simulink library "Kitchen_Lib"  (R2023a)
settings: Solver=VariableStepAuto  StartTime=0.0  StopTime=10.0  RelTol=1e-3  EnableMultiTasking=on
undefined symbols (not defined in the file): Kitc_BusTyp_P, Kitc_BusTypSkyr_C, Kitc_ColrLedColrls_C, Kitc_ColrLedGrn_C, Kitc_ColrLedRed_C, Kitc_ColrLedYlw_C, Kitc_StDgnWtrTank_C, Kitc_StElecPlugScktOffByClmp50_P, Kitc_StsDlyBlink_C, Kitc_StsErrBlink_C, Kitc_StsFctAcvn_P, Kitc_StsInfoBlink_C, Kitc_StsKitchnOffAutoIgOff_P, Kitc_StsKitchnOffBySwt_P, Kitc_StsKitchnOffDoorLockd_P, Kitc_StsKitchnOffIgOff_P, Kitc_StsKitchnOffUv_P, Kitc_StsKitchnOnBySwt_P, Kitc_StsKitchnOnNVM_P, Kitc_StsLedOff_C, Kitc_StsLedOn_C, Kitc_StsLrgCnsAcv_P, Kitc_StTrfrAnSwtInstd_P, Kitc_StTrfrSwtInstd_P, Kitc_TiKitcRefgtrOffDly_P, Kitc_ULowrThdBat_C, Kitc_UUpprThdBat_C, Kitc_ValFalse_C, Kitc_ValPwmFreq2_C, Kitc_ValPwmFreq_C, Kitc_ValTrue_C
libraries: MAN_Library x50, E2E_Lib x3
(part 10 of 13)

== system Kitchen_Lib/Kitchen/100ms/Kitchn/Subsystem1/Subsystem19/Trfr/TurnOnDelay/TurnOnDelayOriginal/RisingEdgeDetection ==
  CLK : Inport
  Constant : Constant  Value=boolean(1)  OutDataTypeStr=boolean
  Data Type Conversion1 : DataTypeConversion  OutDataTypeStr=boolean  SaturateOnIntegerOverflow=off  RndMeth=Floor
  Logical Operator : Logic  AllPortsSameDT=off  OutDataTypeStr=boolean
  Relational Operator : RelationalOperator  Operator=~=  OutDataTypeStr=boolean  InputSameDT=off
  Relational Operator1 : RelationalOperator  Operator===  OutDataTypeStr=boolean  InputSameDT=off
  Unit Delay : UnitDelay  SampleTime=-1  HasFrameUpgradeWarning=on
  Q : Outport
  wires:
  Data Type Conversion1/1 -> Relational Operator1/1, Relational Operator/2, Unit Delay/1
  Constant/1 -> Relational Operator1/2
  Logical Operator/1 -> Q/1
  Relational Operator1/1 -> Logical Operator/2
  Relational Operator/1 -> Logical Operator/1
  Unit Delay/1 -> Relational Operator/1
  CLK/1 -> Data Type Conversion1/1

== system Kitchen_Lib/Kitchen/100ms/Kitchn/Subsystem1/Subsystem19/Trfr/TurnOnDelay/TurnOnDelayOriginal/TimePulseOriginal ==
  TimePulseEnable : Inport
  TimePulseDuration : Inport  Port=2
  CycleTime : Inport  Port=3
  Data Type Conversion1 : DataTypeConversion  OutDataTypeStr=uint32  SaturateOnIntegerOverflow=off  RndMeth=Floor
  Data Type Conversion2 : DataTypeConversion  OutDataTypeStr=boolean  SaturateOnIntegerOverflow=off  RndMeth=Floor
  Delay1 : Delay  DelayLength=1  InitialCondition=0  ExternalReset=Rising
      settings: InputPortMap=u0,r5
  Logical Operator1 : Logic  Operator=NOT  AllPortsSameDT=off  OutDataTypeStr=boolean
  Logical Operator2 : Logic  AllPortsSameDT=off  OutDataTypeStr=boolean
  RisingEdgeDetection : Subsystem  AncestorBlock=MAN_Library/RisingEdgeDetection
  RisingEdgeDetection1 : Subsystem  AncestorBlock=MAN_Library/RisingEdgeDetection
  SR : Subsystem  AncestorBlock=MAN_Library/SR
  TimerCountingUpOriginal : Subsystem  AncestorBlock=MAN_Library/BasicLibrary/TimerCountingUpOriginal
  TimePulseFlag : Outport
  TimePulseExpiredTime : Outport  Port=2
  wires:
  CycleTime/1 -> TimerCountingUpOriginal/4(CycleTime)
  Delay1/1 -> SR/2(R)
  [TimePulseReset] -> TimerCountingUpOriginal/2(TimerReset)
  [TimePulseReset] -> Delay1/2
  RisingEdgeDetection/1(Q) -> SR/1(S), [TimePulseReset]
  Data Type Conversion1/1 -> TimerCountingUpOriginal/3(TimerThreshold)
  Data Type Conversion2/1 -> RisingEdgeDetection/1(CLK)
  Logical Operator1/1 -> Logical Operator2/2
  Logical Operator2/1 -> TimePulseFlag/1
  RisingEdgeDetection1/1(Q) -> Delay1/1
  TimerCountingUpOriginal/1(TimerFlag) -> RisingEdgeDetection1/1(CLK), Logical Operator1/1
  SR/1(Q) -> Logical Operator2/1, TimerCountingUpOriginal/1(TimerEnable)
  TimePulseEnable/1 -> Data Type Conversion2/1
  TimePulseDuration/1 -> Data Type Conversion1/1
  TimerCountingUpOriginal/2(TimerCurrentValue) -> TimePulseExpiredTime/1

== system Kitchen_Lib/Kitchen/100ms/Kitchn/Subsystem1/Subsystem19/WaterTankEmptyDiagnostic/Diagno sticsDebouncing/DiagnosticsDebouncingOriginal/RS ==
  S : Inport
  R : Inport  Port=2
  Constant2 : Constant  Value=boolean(1)  OutDataTypeStr=boolean
  Constant3 : Constant  Value=boolean(0)  OutDataTypeStr=boolean
  Data Type Conversion1 : DataTypeConversion  OutDataTypeStr=boolean  SaturateOnIntegerOverflow=off  RndMeth=Floor
  Data Type Conversion2 : DataTypeConversion  OutDataTypeStr=boolean  SaturateOnIntegerOverflow=off  RndMeth=Floor
  Multiport Switch : MultiPortSwitch  DataPortOrder=Zero-based contiguous  Inputs=2  zeroidx=on  SaturateOnIntegerOverflow=off  InputSameDT=off
  Multiport Switch2 : MultiPortSwitch  DataPortOrder=Zero-based contiguous  Inputs=2  zeroidx=on  SaturateOnIntegerOverflow=off  InputSameDT=off
  Unit Delay : UnitDelay  SampleTime=-1  HasFrameUpgradeWarning=on
  Q : Outport
  wires:
  Data Type Conversion1/1 -> Multiport Switch2/1
  Data Type Conversion2/1 -> Multiport Switch/1
  Multiport Switch2/1 -> Unit Delay/1, Q/1
  Multiport Switch/1 -> Multiport Switch2/2
  Constant3/1 -> Multiport Switch2/3
  R/1 -> Data Type Conversion1/1
  Unit Delay/1 -> Multiport Switch/2
  Constant2/1 -> Multiport Switch/3
  S/1 -> Data Type Conversion2/1

== system Kitchen_Lib/Kitchen/100ms/Kitchn/Subsystem1/Subsystem19/WaterTankEmptyDiagnostic/Diagno sticsDebouncing/DiagnosticsDebouncingOriginal/TurnOffDelayOriginal  ==
  TurnOffDelayEnable : Inport
  TurnOffDelayThreshold : Inport  Port=2
  CycleTime : Inport  Port=3
  Data Type Conversion1 : DataTypeConversion  OutDataTypeStr=uint32  SaturateOnIntegerOverflow=off  RndMeth=Floor
  Data Type Conversion2 : DataTypeConversion  OutDataTypeStr=boolean  SaturateOnIntegerOverflow=off  RndMeth=Floor
  Data Type Conversion3 : DataTypeConversion  OutDataTypeStr=uint32  SaturateOnIntegerOverflow=off  RndMeth=Floor
  FallingEdgeDetection : Subsystem  AncestorBlock=MAN_Library/FallingEdgeDetection
  Logical Operator2 : Logic  Operator=OR  AllPortsSameDT=off  OutDataTypeStr=boolean
  TimePulseOriginal : Subsystem  AncestorBlock=MAN_Library/BasicLibrary/TimePulseOriginal
  TurnOffDelayFlag : Outport
  TurnOffDelayExpiredTime : Outport  Port=2
  wires:
  CycleTime/1 -> TimePulseOriginal/3(CycleTime)
  Data Type Conversion3/1 -> TurnOffDelayExpiredTime/1
  Data Type Conversion1/1 -> TimePulseOriginal/2(TimePulseDuration)
  TurnOffDelayThreshold/1 -> Data Type Conversion1/1
  FallingEdgeDetection/1(Q) -> TimePulseOriginal/1(TimePulseEnable)
  TimePulseOriginal/2(TimePulseExpiredTime) -> Data Type Conversion3/1
  Logical Operator2/1 -> TurnOffDelayFlag/1
  TimePulseOriginal/1(TimePulseFlag) -> Logical Operator2/2
  Data Type Conversion2/1 -> FallingEdgeDetection/1(CLK), Logical Operator2/1
  TurnOffDelayEnable/1 -> Data Type Conversion2/1

== system Kitchen_Lib/Kitchen/100ms/Kitchn/Subsystem1/Subsystem19/WaterTankEmptyDiagnostic/Diagno sticsDebouncing/DiagnosticsDebouncingOriginal/TurnOnDelayOriginal ==
  TurnOnDelayEnable : Inport
  TurnOnDelayThreshold : Inport  Port=2
  CycleTime : Inport  Port=3
  Data Type Conversion1 : DataTypeConversion  OutDataTypeStr=uint32  SaturateOnIntegerOverflow=off  RndMeth=Floor
  Data Type Conversion2 : DataTypeConversion  OutDataTypeStr=boolean  SaturateOnIntegerOverflow=off  RndMeth=Floor
  Logical Operator1 : Logic  Operator=NOT  AllPortsSameDT=off  OutDataTypeStr=boolean
  Logical Operator2 : Logic  AllPortsSameDT=off  OutDataTypeStr=boolean
  RisingEdgeDetection : Subsystem  AncestorBlock=MAN_Library/RisingEdgeDetection
  TimePulseOriginal : Subsystem  AncestorBlock=MAN_Library/BasicLibrary/TimePulseOriginal
  TurnOnDelayFlag : Outport
  TurnOnDelayExpiredTime : Outport  Port=2
  wires:
  CycleTime/1 -> TimePulseOriginal/3(CycleTime)
  Logical Operator2/1 -> TurnOnDelayFlag/1
  TimePulseOriginal/1(TimePulseFlag) -> Logical Operator1/1
  Logical Operator1/1 -> Logical Operator2/2
  TimePulseOriginal/2(TimePulseExpiredTime) -> TurnOnDelayExpiredTime/1
  RisingEdgeDetection/1(Q) -> TimePulseOriginal/1(TimePulseEnable)
  Data Type Conversion1/1 -> TimePulseOriginal/2(TimePulseDuration)
  TurnOnDelayThreshold/1 -> Data Type Conversion1/1
  TurnOnDelayEnable/1 -> Data Type Conversion2/1
  Data Type Conversion2/1 -> RisingEdgeDetection/1(CLK), Logical Operator2/1

== system Kitchen_Lib/Kitchen/100ms/Kitchn/Subsystem1/Subsystem19/WaterTankEmptyDiagnostic/TurnOffDelay/TurnOffDelayOriginal/FallingEdgeDetection ==
  CLK : Inport
  Constant : Constant  Value=boolean(0)  OutDataTypeStr=boolean
  Data Type Conversion1 : DataTypeConversion  OutDataTypeStr=boolean  SaturateOnIntegerOverflow=off  RndMeth=Floor
  Logical Operator1 : Logic  AllPortsSameDT=off  OutDataTypeStr=boolean
  Relational Operator2 : RelationalOperator  Operator=~=  OutDataTypeStr=boolean  InputSameDT=off
  Relational Operator3 : RelationalOperator  Operator===  OutDataTypeStr=boolean  InputSameDT=off
  Unit Delay1 : UnitDelay  SampleTime=-1  HasFrameUpgradeWarning=on
  Q : Outport
  wires:
  Data Type Conversion1/1 -> Unit Delay1/1, Relational Operator2/2, Relational Operator3/1
  Constant/1 -> Relational Operator3/2
  CLK/1 -> Data Type Conversion1/1
  Logical Operator1/1 -> Q/1
  Relational Operator3/1 -> Logical Operator1/2
  Relational Operator2/1 -> Logical Operator1/1
  Unit Delay1/1 -> Relational Operator2/1

== system Kitchen_Lib/Kitchen/100ms/Kitchn/Subsystem1/Subsystem19/WaterTankEmptyDiagnostic/TurnOffDelay/TurnOffDelayOriginal/TimePulseOriginal ==
  TimePulseEnable : Inport
  TimePulseDuration : Inport  Port=2
  CycleTime : Inport  Port=3
  Data Type Conversion1 : DataTypeConversion  OutDataTypeStr=uint32  SaturateOnIntegerOverflow=off  RndMeth=Floor
  Data Type Conversion2 : DataTypeConversion  OutDataTypeStr=boolean  SaturateOnIntegerOverflow=off  RndMeth=Floor
  Delay1 : Delay  DelayLength=1  InitialCondition=0  ExternalReset=Rising
      settings: InputPortMap=u0,r5
  Logical Operator1 : Logic  Operator=NOT  AllPortsSameDT=off  OutDataTypeStr=boolean
  Logical Operator2 : Logic  AllPortsSameDT=off  OutDataTypeStr=boolean
  RisingEdgeDetection : Subsystem  AncestorBlock=MAN_Library/RisingEdgeDetection
  RisingEdgeDetection1 : Subsystem  AncestorBlock=MAN_Library/RisingEdgeDetection
  SR : Subsystem  AncestorBlock=MAN_Library/SR
  TimerCountingUpOriginal : Subsystem  AncestorBlock=MAN_Library/BasicLibrary/TimerCountingUpOriginal
  TimePulseFlag : Outport
  TimePulseExpiredTime : Outport  Port=2
  wires:
  CycleTime/1 -> TimerCountingUpOriginal/4(CycleTime)
  Delay1/1 -> SR/2(R)
  [TimePulseReset] -> TimerCountingUpOriginal/2(TimerReset)
  [TimePulseReset] -> Delay1/2
  RisingEdgeDetection/1(Q) -> SR/1(S), [TimePulseReset]
  Data Type Conversion1/1 -> TimerCountingUpOriginal/3(TimerThreshold)
  Data Type Conversion2/1 -> RisingEdgeDetection/1(CLK)
  Logical Operator1/1 -> Logical Operator2/2
  Logical Operator2/1 -> TimePulseFlag/1
  RisingEdgeDetection1/1(Q) -> Delay1/1
  TimerCountingUpOriginal/1(TimerFlag) -> RisingEdgeDetection1/1(CLK), Logical Operator1/1
  SR/1(Q) -> Logical Operator2/1, TimerCountingUpOriginal/1(TimerEnable)
  TimePulseEnable/1 -> Data Type Conversion2/1
  TimePulseDuration/1 -> Data Type Conversion1/1
  TimerCountingUpOriginal/2(TimerCurrentValue) -> TimePulseExpiredTime/1

== system Kitchen_Lib/Kitchen/100ms/Kitchn/Subsystem1/Subsystem16/001_KitchnCtl/002_FlipFlop/KSW-KitchenControl/KSW_Battery/BatteryVoltageUnder22.7V ==
  Kitchn_On : Inport
  EngOrAddlBat : Inport  Port=2
  "GW_Ubat " : Inport  Port=3
  Constant : Constant  Value=Kitc_StsLrgCnsAcv_P
  Constant2 : Constant  Value=Kitc_ULowrThdBat_C
  Data Store Read : DataStoreRead  DataStoreName=Kitc_StsLrgCnsAcvNv  IndexOptions=Index vector (dialog)  Indices=1  OutputSizes=1
  Data Type Conversion : DataTypeConversion  OutDataTypeStr=boolean  SaturateOnIntegerOverflow=off  RndMeth=Floor
  Logical Operator1 : Logic  Operator=NOT  Inputs=4  AllPortsSameDT=off  OutDataTypeStr=boolean
  Logical Operator2 : Logic  Inputs=4  AllPortsSameDT=off  OutDataTypeStr=boolean
  Relational Operator1 : RelationalOperator  Operator=<=  OutDataTypeStr=boolean  InputSameDT=off
  Switch : Switch  Criteria=u2 ~= 0  SaturateOnIntegerOverflow=off  InputSameDT=off
  BatUUnder22.7V : Outport
  wires:
  Data Type Conversion/1 -> Switch/2
  Constant/1 -> Switch/3
  Data Store Read/1 -> Switch/1, Data Type Conversion/1
  Logical Operator2/1 -> BatUUnder22.7V/1
  EngOrAddlBat/1 -> Logical Operator1/1
  "GW_Ubat "/1 -> Relational Operator1/1
  Constant2/1 -> Relational Operator1/2
  Relational Operator1/1 -> Logical Operator2/4
  Logical Operator1/1 -> Logical Operator2/1
  Switch/1 -> Logical Operator2/3
  Kitchn_On/1 -> Logical Operator2/2

== system Kitchen_Lib/Kitchen/100ms/Kitchn/Subsystem1/Subsystem16/001_KitchnCtl/002_FlipFlop/KSW-KitchenControl/KSW_Battery/BatteryVoltageUnder23V ==
  GW_Ubat : Inport
  EngOrAddlBat : Inport  Port=2
  Kitchn_On : Inport  Port=3
  Kitc_StsHostsCallAcv : Inport  Port=4
  Constant : Constant  Value=Kitc_StsLrgCnsAcv_P
  Constant1 : Constant  Value=Kitc_UUpprThdBat_C
  "Constant3  " : MAN_Library/TimeConstant  hours=0  minutes=0  seconds=10  miliseconds=0
  "Constant4  " : MAN_Library/TimeConstant  hours=0  minutes=10  seconds=0  miliseconds=0
  "Constant6  " : MAN_Library/TimeConstant  hours=0  minutes=0  seconds=0  miliseconds=500
  Data Store Read : DataStoreRead  DataStoreName=Kitc_StsLrgCnsAcvNv  IndexOptions=Index vector (dialog)  Indices=1  OutputSizes=1
  Data Type Conversion : DataTypeConversion  OutDataTypeStr=boolean  SaturateOnIntegerOverflow=off  RndMeth=Floor
  Logical Operator15 : Logic  Operator=OR  AllPortsSameDT=off  OutDataTypeStr=boolean
  Logical Operator16 : Logic  Operator=NOT  Inputs=4  AllPortsSameDT=off  OutDataTypeStr=boolean
  Logical Operator3 : Logic  Inputs=4  AllPortsSameDT=off  OutDataTypeStr=boolean
  Logical Operator4 : Logic  Operator=NOT  Inputs=4  AllPortsSameDT=off  OutDataTypeStr=boolean
  Relational Operator : RelationalOperator  Operator=<=  OutDataTypeStr=boolean  InputSameDT=off
  Switch : Switch  Criteria=u2 ~= 0  SaturateOnIntegerOverflow=off  InputSameDT=off
  Terminator : Terminator
  Terminator1 : Terminator
  Terminator2 : Terminator
  TimePulse : MAN_Library/TimePulse  CycleTime=Cycle Time: 10 Ms
  TimePulse1 : MAN_Library/TimePulse  CycleTime=Cycle Time: 10 Ms
  TurnOffDelay : MAN_Library/TurnOffDelay  CycleTime=Cycle Time: 10 Ms
  LrgCnsOff : Outport
  Kitc_WarnLrgCns : Outport  Port=2
  Kitc_StBuzRe : Outport  Port=3
  wires:
  Data Type Conversion/1 -> Switch/2
  Constant/1 -> Switch/3
  Data Store Read/1 -> Switch/1, Data Type Conversion/1
  Switch/1 -> Logical Operator3/3
  Constant1/1 -> Relational Operator/2
  Relational Operator/1 -> Logical Operator3/4
  Kitchn_On/1 -> Logical Operator3/2
  Logical Operator16/1 -> Logical Operator3/1
  EngOrAddlBat/1 -> Logical Operator16/1
  GW_Ubat/1 -> Relational Operator/1
  "Constant3  "/1 -> TimePulse/2
  TimePulse/1 -> Kitc_WarnLrgCns/1, Logical Operator15/1
  "Constant4  "/1 -> TurnOffDelay/2
  Logical Operator4/1 -> TurnOffDelay/1
  TurnOffDelay/1 -> LrgCnsOff/1
  Kitc_StsHostsCallAcv/1 -> TimePulse1/1
  Logical Operator15/1 -> Kitc_StBuzRe/1
  "Constant6  "/1 -> TimePulse1/2
  TimePulse1/1 -> Logical Operator15/2
  TurnOffDelay/2 -> Terminator/1
  TimePulse/2 -> Terminator1/1
  TimePulse1/2 -> Terminator2/1
  Logical Operator3/1 -> Logical Operator4/1, TimePulse/1

== system Kitchen_Lib/Kitchen/100ms/Kitchn/Subsystem1/Subsystem16/001_KitchnCtl/002_FlipFlop/KSW-KitchenControl/KSW_Battery/KitchenActivation ==
  note: Large Comsp
  "GW_StClmp50Off3Sec " : Inport
  "GW_StUvTopPrio " : Inport  Port=2
  "GW_ModeExbn " : Inport  Port=3
  CLS_StDoorLockdOutd : Inport  Port=4
  BatUUnder22.7V : Inport  Port=5
  LrgCnsOff : Inport  Port=6
  Kitchn_On : Inport  Port=7
  GW_StClmp15 : Inport  Port=8
  EngOrAddlBat : Inport  Port=9
  Constant : Constant  Value=Kitc_StsLrgCnsAcv_P
  Data Store Read : DataStoreRead  DataStoreName=Kitc_StsLrgCnsAcvNv  IndexOptions=Index vector (dialog)  Indices=1  OutputSizes=1
  Data Type Conversion : DataTypeConversion  OutDataTypeStr=boolean  SaturateOnIntegerOverflow=off  RndMeth=Floor
  Logical Operator{1,9..12} (5 alike) : Logic  Operator=NOT  Inputs=4  AllPortsSameDT=off  OutDataTypeStr=boolean
  Logical Operator13 : Logic  Operator=OR  AllPortsSameDT=off  OutDataTypeStr=boolean
  Logical Operator14 : Logic  AllPortsSameDT=off  OutDataTypeStr=boolean
  Logical Operator5 : Logic  Operator=OR  AllPortsSameDT=off  OutDataTypeStr=boolean
  Logical Operator6 : Logic  Inputs=3  AllPortsSameDT=off  OutDataTypeStr=boolean
  Logical Operator7 : Logic  Inputs=9  AllPortsSameDT=off  OutDataTypeStr=boolean
  Switch : Switch  Criteria=u2 ~= 0  SaturateOnIntegerOverflow=off  InputSameDT=off
  KitchnAcv : Outport
  LrgCnsEna : Outport  Port=2
  LrgCns : Outport  Port=3
  wires:
  Data Type Conversion/1 -> Switch/2
  Constant/1 -> Switch/3
  Data Store Read/1 -> Switch/1, Data Type Conversion/1
  Logical Operator13/1 -> KitchnAcv/1
  Logical Operator6/1 -> Logical Operator5/2
  Logical Operator5/1 -> Logical Operator14/2, LrgCns/1, Logical Operator13/1
  Logical Operator11/1 -> Logical Operator14/1, Logical Operator7/1
  Logical Operator14/1 -> LrgCnsEna/1
  Logical Operator9/1 -> Logical Operator7/2
  "GW_StUvTopPrio "/1 -> Logical Operator9/1
  Logical Operator12/1 -> Logical Operator7/4
  Switch/1 -> Logical Operator7/5
  Logical Operator7/1 -> Logical Operator5/1
  "GW_ModeExbn "/1 -> Logical Operator10/1
  Logical Operator10/1 -> Logical Operator7/3
  CLS_StDoorLockdOutd/1 -> Logical Operator12/1
  "GW_StClmp50Off3Sec "/1 -> Logical Operator11/1
  GW_StClmp15/1 -> Logical Operator7/8, Logical Operator6/2
  BatUUnder22.7V/1 -> Logical Operator1/1
  Kitchn_On/1 -> Logical Operator6/1, [Kitchn_On], Logical Operator7/9
  LrgCnsOff/1 -> Logical Operator7/7
  EngOrAddlBat/1 -> Logical Operator6/3
  Logical Operator1/1 -> Logical Operator7/6
  [Kitchn_On] -> Logical Operator13/2

== system Kitchen_Lib/Kitchen/100ms/Kitchn/Subsystem1/Subsystem16/001_KitchnCtl/002_FlipFlop/KitchenEnable/KitchenOnNVM/NVM ==
  KitchnOffBySwt : Inport
  HostsSideBotmBtn_OFF : Inport  Port=2
  "GW_StStrtNew " : Inport  Port=3
  Kitc_ModeKitcNv : Inport  Port=4
  Kitchn_On : Inport  Port=5
  GW_StClmp15 : Inport  Port=6
  Data Store Write : DataStoreWrite  DataStoreName=Kitc_ModeKitcNv  IndexOptions=Index vector (dialog)  Indices=1  OutputSizes=1
  Logical Operator41 : Logic  Operator=OR  Inputs=3  AllPortsSameDT=off  OutDataTypeStr=boolean
  Logical Operator{42..43,46,48} (4 alike) : Logic  AllPortsSameDT=off  OutDataTypeStr=boolean
  Logical Operator44 : Logic  Inputs=4  AllPortsSameDT=off  OutDataTypeStr=boolean
  Logical Operator45 : Logic  Operator=NOT  Inputs=4  AllPortsSameDT=off  OutDataTypeStr=boolean
  Logical Operator47 : Logic  Operator=NOT  Inputs=4  AllPortsSameDT=off  OutDataTypeStr=boolean
  Logical Operator49 : Logic  Operator=NOT  Inputs=4  AllPortsSameDT=off  OutDataTypeStr=boolean
  RisingEdgeDetection1 : MAN_Library/RisingEdgeDetection
  RisingEdgeDetection2 : MAN_Library/RisingEdgeDetection
  wires:
  Logical Operator48/1 -> Logical Operator49/1
  RisingEdgeDetection1/1 -> Logical Operator42/1
  Logical Operator49/1 -> Logical Operator44/4
  Logical Operator44/1 -> Data Store Write/1
  Kitchn_On/1 -> Logical Operator42/2, RisingEdgeDetection2/1
  Logical Operator45/1 -> Logical Operator44/2
  Logical Operator41/1 -> Logical Operator44/1
  Kitc_ModeKitcNv/1 -> Logical Operator41/1
  RisingEdgeDetection2/1 -> Logical Operator43/1
  Logical Operator46/1 -> Logical Operator47/1
  Logical Operator43/1 -> Logical Operator41/3
  Logical Operator42/1 -> Logical Operator41/2
  Logical Operator47/1 -> Logical Operator44/3
  GW_StClmp15/1 -> RisingEdgeDetection1/1, Logical Operator48/1, Logical Operator46/1, Logical Operator43/2
  KitchnOffBySwt/1 -> Logical Operator46/2
  HostsSideBotmBtn_OFF/1 -> Logical Operator48/2
  "GW_StStrtNew "/1 -> Logical Operator45/1

== system Kitchen_Lib/Kitchen/100ms/Kitchn/Subsystem1/Subsystem16/001_KitchnCtl/002_FlipFlop/KitchenEnable/Subsystem/RS ==
  S : Inport
  R : Inport  Port=2
  Constant2 : Constant  Value=boolean(1)  OutDataTypeStr=boolean
  Constant3 : Constant  Value=boolean(0)  OutDataTypeStr=boolean
  Data Type Conversion1 : DataTypeConversion  OutDataTypeStr=boolean  SaturateOnIntegerOverflow=off  RndMeth=Floor
  Data Type Conversion2 : DataTypeConversion  OutDataTypeStr=boolean  SaturateOnIntegerOverflow=off  RndMeth=Floor
  Multiport Switch : MultiPortSwitch  DataPortOrder=Zero-based contiguous  Inputs=2  zeroidx=on  SaturateOnIntegerOverflow=off  InputSameDT=off
  Multiport Switch2 : MultiPortSwitch  DataPortOrder=Zero-based contiguous  Inputs=2  zeroidx=on  SaturateOnIntegerOverflow=off  InputSameDT=off
  Unit Delay : UnitDelay  SampleTime=-1  HasFrameUpgradeWarning=on
  Q : Outport
  wires:
  Data Type Conversion1/1 -> Multiport Switch2/1
  Data Type Conversion2/1 -> Multiport Switch/1
  Multiport Switch2/1 -> Unit Delay/1, Q/1
  Multiport Switch/1 -> Multiport Switch2/2
  Constant3/1 -> Multiport Switch2/3
  R/1 -> Data Type Conversion1/1
  Unit Delay/1 -> Multiport Switch/2
  Constant2/1 -> Multiport Switch/3
  S/1 -> Data Type Conversion2/1

== system Kitchen_Lib/Kitchen/100ms/Kitchn/Subsystem1/Subsystem16/001_KitchnCtl/002_FlipFlop/KitchenEnable/Subsystem/RisingEdgeDetection ==
  CLK : Inport
  Constant : Constant  Value=boolean(1)  OutDataTypeStr=boolean
  Data Type Conversion1 : DataTypeConversion  OutDataTypeStr=boolean  SaturateOnIntegerOverflow=off  RndMeth=Floor
  Logical Operator : Logic  AllPortsSameDT=off  OutDataTypeStr=boolean
  Relational Operator : RelationalOperator  Operator=~=  OutDataTypeStr=boolean  InputSameDT=off
  Relational Operator1 : RelationalOperator  Operator===  OutDataTypeStr=boolean  InputSameDT=off
  Unit Delay : UnitDelay  SampleTime=-1  HasFrameUpgradeWarning=on
  Q : Outport
  wires:
  Data Type Conversion1/1 -> Relational Operator1/1, Relational Operator/2, Unit Delay/1
  Constant/1 -> Relational Operator1/2
  Logical Operator/1 -> Q/1
  Relational Operator1/1 -> Logical Operator/2
  Relational Operator/1 -> Logical Operator/1
  Unit Delay/1 -> Relational Operator/1
  CLK/1 -> Data Type Conversion1/1

== system Kitchen_Lib/Kitchen/100ms/Kitchn/Subsystem1/Subsystem16/001_KitchnCtl/002_FlipFlop/KitchenEnable/Subsystem/StateChangePulse ==
  note: This function replaces '2k+1 XOR' block to detect changes.
  IN : Inport
  Data Type Conversion1 : DataTypeConversion  OutDataTypeStr=boolean  SaturateOnIntegerOverflow=off  RndMeth=Floor
  Data Type Conversion2 : DataTypeConversion  Commented=on  OutDataTypeStr=boolean  SaturateOnIntegerOverflow=off  RndMeth=Floor
  Ground : Ground  Commented=on
  Logical Operator17 : Logic  Operator=XOR  AllPortsSameDT=off  OutDataTypeStr=boolean
  Relational Operator : RelationalOperator  Commented=on  Operator=~=  OutDataTypeStr=boolean  InputSameDT=off
  Terminator : Terminator  Commented=on
  Unit Delay : UnitDelay  SampleTime=-1  HasFrameUpgradeWarning=on
  Unit Delay1 : UnitDelay  Commented=on  SampleTime=-1  HasFrameUpgradeWarning=on
  OUT : Outport
  wires:
  Unit Delay1/1 -> Relational Operator/1
  IN/1 -> Data Type Conversion1/1
  Ground/1 -> Data Type Conversion2/1
  Relational Operator/1 -> Terminator/1
  Data Type Conversion2/1 -> Unit Delay1/1, Relational Operator/2
  Data Type Conversion1/1 -> Logical Operator17/1
  Unit Delay/1 -> Logical Operator17/2
  Logical Operator17/1 -> Unit Delay/1, OUT/1

== system Kitchen_Lib/Kitchen/100ms/Kitchn/Subsystem1/Subsystem16/001_KitchnCtl/002_FlipFlop/KitchenEnable/Subsystem/TimeConstant ==
  Constant11 : Constant  Value=uint32(hours)  OutDataTypeStr=uint32
  Constant12 : Constant  Value=uint32(minutes)  OutDataTypeStr=uint32
  Constant13 : Constant  Value=uint32(miliseconds)  OutDataTypeStr=uint32
  Constant14 : Constant  Value=uint32(60)  OutDataTypeStr=uint32
  Constant15 : Constant  Value=uint32(1000)  OutDataTypeStr=uint32
  Constant16 : Constant  Value=uint32(seconds)  OutDataTypeStr=uint32
  Constant17 : Constant  Value=uint32(1000)  OutDataTypeStr=uint32
  Constant7 : Constant  Value=uint32(60)  OutDataTypeStr=uint32
  Constant8 : Constant  Value=uint32(60)  OutDataTypeStr=uint32
  Constant9 : Constant  Value=uint32(1000)  OutDataTypeStr=uint32
  Data Type Conversion{1..2,4..8,13..19} (14 alike) : DataTypeConversion  OutDataTypeStr=uint32  SaturateOnIntegerOverflow=off  RndMeth=Floor
  Product1 : Product  Inputs=4  OutDataTypeStr=uint32
  Product2 : Product  Inputs=3  OutDataTypeStr=uint32
  Product4 : Product  OutDataTypeStr=uint32
  Sum1 : Sum  Inputs=++++  AccumDataTypeStr=uint32
  time : Outport
  wires:
  Data Type Conversion8/1 -> Sum1/4
  Data Type Conversion7/1 -> Sum1/3
  Data Type Conversion6/1 -> Sum1/2
  Data Type Conversion4/1 -> Sum1/1
  Constant13/1 -> Data Type Conversion8/1
  Data Type Conversion2/1 -> Product2/3
  Data Type Conversion1/1 -> Product4/2
  Product4/1 -> Data Type Conversion7/1
  Product2/1 -> Data Type Conversion6/1
  Product1/1 -> Data Type Conversion4/1
  Constant16/1 -> Data Type Conversion1/1
  Data Type Conversion19/1 -> Product4/1
  Constant17/1 -> Data Type Conversion19/1
  Data Type Conversion18/1 -> Product2/2
  Constant15/1 -> Data Type Conversion18/1
  Data Type Conversion17/1 -> Product2/1
  Constant14/1 -> Data Type Conversion17/1
  Constant12/1 -> Data Type Conversion2/1
  Data Type Conversion16/1 -> Product1/4
  Constant11/1 -> Data Type Conversion16/1
  Data Type Conversion15/1 -> Product1/3
  Constant9/1 -> Data Type Conversion15/1
  Data Type Conversion14/1 -> Product1/2
  Constant8/1 -> Data Type Conversion14/1
  Data Type Conversion13/1 -> Product1/1
  Constant7/1 -> Data Type Conversion13/1
  Data Type Conversion5/1 -> time/1
  Sum1/1 -> Data Type Conversion5/1  "time"

== system Kitchen_Lib/Kitchen/100ms/Kitchn/Subsystem1/Subsystem16/001_KitchnCtl/002_FlipFlop/KitchenEnable/Subsystem/TurnOnDelay ==
  TurnOnDelayEnable : Inport
  TurnOnDelayThreshold : Inport  Port=2
  Constant10 : Constant  Value=uint32(CycleTime)  OutDataTypeStr=uint32
  Constant16 : Constant  Value=uint32(1)  OutDataTypeStr=uint32
  Constant17 : Constant  Value=uint32(10)  OutDataTypeStr=uint32
  Constant18 : Constant  Value=uint32(100)  OutDataTypeStr=uint32
  Constant19 : Constant  Value=uint32(1000)  OutDataTypeStr=uint32
  Multiport Switch4 : MultiPortSwitch  Inputs=4  SaturateOnIntegerOverflow=off  InputSameDT=off
  TurnOnDelayOriginal : Subsystem  AncestorBlock=MAN_Library/BasicLibrary/TurnOnDelayOriginal
  TurnOnDelayFlag : Outport
  TurnOnDelayExpiredTime : Outport  Port=2
  wires:
  TurnOnDelayOriginal/1(TurnOnDelayFlag) -> TurnOnDelayFlag/1
  TurnOnDelayOriginal/2(TurnOnDelayExpiredTime) -> TurnOnDelayExpiredTime/1
  TurnOnDelayThreshold/1 -> TurnOnDelayOriginal/2(TurnOnDelayThreshold)
  TurnOnDelayEnable/1 -> TurnOnDelayOriginal/1(TurnOnDelayEnable)
  Constant19/1 -> Multiport Switch4/5
  Constant18/1 -> Multiport Switch4/4
  Constant17/1 -> Multiport Switch4/3
  Constant16/1 -> Multiport Switch4/2
  Constant10/1 -> Multiport Switch4/1
  Multiport Switch4/1 -> TurnOnDelayOriginal/3(CycleTime)

== system Kitchen_Lib/Kitchen/100ms/Kitchn/Subsystem1/Subsystem19/KSW_Battery/BatteryVoltageUnder23V/TimePulse/TimePulseOriginal/RisingEdgeDetection ==
  CLK : Inport
  Constant : Constant  Value=boolean(1)  OutDataTypeStr=boolean
  Data Type Conversion1 : DataTypeConversion  OutDataTypeStr=boolean  SaturateOnIntegerOverflow=off  RndMeth=Floor
  Logical Operator : Logic  AllPortsSameDT=off  OutDataTypeStr=boolean
  Relational Operator : RelationalOperator  Operator=~=  OutDataTypeStr=boolean  InputSameDT=off
  Relational Operator1 : RelationalOperator  Operator===  OutDataTypeStr=boolean  InputSameDT=off
  Unit Delay : UnitDelay  SampleTime=-1  HasFrameUpgradeWarning=on
  Q : Outport
  wires:
  Data Type Conversion1/1 -> Relational Operator1/1, Relational Operator/2, Unit Delay/1
  Constant/1 -> Relational Operator1/2
  Logical Operator/1 -> Q/1
  Relational Operator1/1 -> Logical Operator/2
  Relational Operator/1 -> Logical Operator/1
  Unit Delay/1 -> Relational Operator/1
  CLK/1 -> Data Type Conversion1/1

== system Kitchen_Lib/Kitchen/100ms/Kitchn/Subsystem1/Subsystem19/KSW_Battery/BatteryVoltageUnder23V/TimePulse/TimePulseOriginal/RisingEdgeDetection1 ==
  CLK : Inport
  Constant : Constant  Value=boolean(1)  OutDataTypeStr=boolean
  Data Type Conversion1 : DataTypeConversion  OutDataTypeStr=boolean  SaturateOnIntegerOverflow=off  RndMeth=Floor
  Logical Operator : Logic  AllPortsSameDT=off  OutDataTypeStr=boolean
  Relational Operator : RelationalOperator  Operator=~=  OutDataTypeStr=boolean  InputSameDT=off
  Relational Operator1 : RelationalOperator  Operator===  OutDataTypeStr=boolean  InputSameDT=off
  Unit Delay : UnitDelay  SampleTime=-1  HasFrameUpgradeWarning=on
  Q : Outport
  wires:
  Data Type Conversion1/1 -> Relational Operator1/1, Relational Operator/2, Unit Delay/1
  Constant/1 -> Relational Operator1/2
  Logical Operator/1 -> Q/1
  Relational Operator1/1 -> Logical Operator/2
  Relational Operator/1 -> Logical Operator/1
  Unit Delay/1 -> Relational Operator/1
  CLK/1 -> Data Type Conversion1/1

== system Kitchen_Lib/Kitchen/100ms/Kitchn/Subsystem1/Subsystem19/KSW_Battery/BatteryVoltageUnder23V/TimePulse/TimePulseOriginal/SR ==
  S : Inport
  R : Inport  Port=2
  Constant1 : Constant  Value=boolean(1)  OutDataTypeStr=boolean
  Constant3 : Constant  Value=boolean(0)  OutDataTypeStr=boolean
  Data Type Conversion1 : DataTypeConversion  OutDataTypeStr=boolean  SaturateOnIntegerOverflow=off  RndMeth=Floor
  Data Type Conversion2 : DataTypeConversion  OutDataTypeStr=boolean  SaturateOnIntegerOverflow=off  RndMeth=Floor
  Multiport Switch : MultiPortSwitch  DataPortOrder=Zero-based contiguous  Inputs=2  zeroidx=on  SaturateOnIntegerOverflow=off  InputSameDT=off
  Multiport Switch1 : MultiPortSwitch  DataPortOrder=Zero-based contiguous  Inputs=2  zeroidx=on  SaturateOnIntegerOverflow=off  InputSameDT=off
  Unit Delay : UnitDelay  SampleTime=-1  HasFrameUpgradeWarning=on
  Q : Outport
  wires:
  Data Type Conversion2/1 -> Multiport Switch/1
  Data Type Conversion1/1 -> Multiport Switch1/1
  Constant3/1 -> Multiport Switch1/3
  Multiport Switch/1 -> Unit Delay/1, Q/1
  Unit Delay/1 -> Multiport Switch1/2
  R/1 -> Data Type Conversion1/1
  Multiport Switch1/1 -> Multiport Switch/2
  Constant1/1 -> Multiport Switch/3
  S/1 -> Data Type Conversion2/1

== system Kitchen_Lib/Kitchen/100ms/Kitchn/Subsystem1/Subsystem19/KSW_Battery/BatteryVoltageUnder23V/TimePulse/TimePulseOriginal/TimerCountingUpOriginal ==
  TimerEnable : Inport
  TimerReset : Inport  Port=2
  TimerThreshold : Inport  Port=3
  CycleTime : Inport  Port=4
  Data Type Conversion2 : DataTypeConversion  OutDataTypeStr=boolean  SaturateOnIntegerOverflow=off  RndMeth=Floor
  Data Type Conversion4 : DataTypeConversion  OutDataTypeStr=uint32  SaturateOnIntegerOverflow=off  RndMeth=Floor
  Data Type Conversion5 : DataTypeConversion  OutDataTypeStr=uint32  SaturateOnIntegerOverflow=off  RndMeth=Floor
  Data Type Conversion6 : DataTypeConversion  OutDataTypeStr=uint32  SaturateOnIntegerOverflow=off  RndMeth=Floor
  Data Type Conversion7 : DataTypeConversion  OutDataTypeStr=boolean  SaturateOnIntegerOverflow=off  RndMeth=Floor
  Delay : Delay  DelayLength=1  InitialCondition=0  ExternalReset=Rising
      settings: InputPortMap=u0,r5
  Delay1 : Delay  DelayLength=1  InitialCondition=0
  Logical Operator1 : Logic  Operator=NOT  AllPortsSameDT=off  OutDataTypeStr=boolean
  Logical Operator2 : Logic  AllPortsSameDT=off  OutDataTypeStr=boolean
  Logical Operator3 : Logic  Operator=OR  AllPortsSameDT=off  OutDataTypeStr=boolean
  Multiport Switch : MultiPortSwitch  DataPortOrder=Zero-based contiguous  Inputs=2  zeroidx=on  SaturateOnIntegerOverflow=off  InputSameDT=off
  Multiport Switch1 : MultiPortSwitch  DataPortOrder=Zero-based contiguous  Inputs=2  zeroidx=on  SaturateOnIntegerOverflow=off  InputSameDT=off
  Multiport Switch2 : MultiPortSwitch  DataPortOrder=Zero-based contiguous  Inputs=2  zeroidx=on  SaturateOnIntegerOverflow=off  InputSameDT=off
  Relational Operator : RelationalOperator  OutDataTypeStr=boolean  InputSameDT=off
  Relational Operator1 : RelationalOperator  Operator===  OutDataTypeStr=boolean  InputSameDT=off
  RisingEdgeDetection : Subsystem  AncestorBlock=MAN_Library/RisingEdgeDetection
  StartValue_ms1 : Constant  Value=uint32(4294967295)  OutDataTypeStr=uint32
  StartValue_ms2 : Constant  Value=uint32(4294967295)  OutDataTypeStr=uint32
  StartValue_ms3 : Constant  Value=uint32(0)  OutDataTypeStr=uint32
  StartValue_ms5 : Constant  Value=uint32(4294967295)  OutDataTypeStr=uint32
  Sum : Sum
  U32_Saturation : Subsystem  AncestorBlock=MAN_Library/U32_Saturation
  TimerFlag : Outport
  TimerCurrentValue : Outport  Port=2
  wires:
  CycleTime/1 -> Data Type Conversion4/1
  Data Type Conversion2/1 -> Logical Operator3/1
  RisingEdgeDetection/1(Q) -> Logical Operator3/2
  TimerReset/1 -> Data Type Conversion2/1
  TimerEnable/1 -> Data Type Conversion7/1
  Data Type Conversion6/1 -> Relational Operator/2
  Data Type Conversion4/1 -> Sum/2
  StartValue_ms3/1 -> U32_Saturation/3(LowerLimit), Multiport Switch/3
  Multiport Switch2/1 -> U32_Saturation/2(IN)
  Sum/1 -> Multiport Switch2/2
  StartValue_ms2/1 -> Multiport Switch2/3
  Relational Operator1/1 -> Multiport Switch2/1
  Delay/1 -> Multiport Switch1/2, Relational Operator1/1, Sum/1
  StartValue_ms5/1 -> Relational Operator1/2
  Logical Operator3/1 -> Multiport Switch/1, [ResetTimer_BOOL]
  StartValue_ms1/1 -> U32_Saturation/1(UpperLimit)
  Delay1/1 -> Logical Operator1/1
  U32_Saturation/1(OUT) -> Multiport Switch1/3
  Logical Operator1/1 -> Logical Operator2/2
  Logical Operator2/1 -> Multiport Switch1/1
  Data Type Conversion5/1 -> TimerCurrentValue/1, Delay/1, Relational Operator/1
  Data Type Conversion7/1 -> Logical Operator2/1, RisingEdgeDetection/1(CLK)
  Multiport Switch/1 -> Data Type Conversion5/1
  Relational Operator/1 -> TimerFlag/1, Delay1/1
  Multiport Switch1/1 -> Multiport Switch/2
  TimerThreshold/1 -> Data Type Conversion6/1
  [ResetTimer_BOOL] -> Delay/2

== system Kitchen_Lib/Kitchen/100ms/Kitchn/Subsystem1/Subsystem19/KSW_Battery/BatteryVoltageUnder23V/TimePulse1/TimePulseOriginal/RisingEdgeDetection ==
  CLK : Inport
  Constant : Constant  Value=boolean(1)  OutDataTypeStr=boolean
  Data Type Conversion1 : DataTypeConversion  OutDataTypeStr=boolean  SaturateOnIntegerOverflow=off  RndMeth=Floor
  Logical Operator : Logic  AllPortsSameDT=off  OutDataTypeStr=boolean
  Relational Operator : RelationalOperator  Operator=~=  OutDataTypeStr=boolean  InputSameDT=off
  Relational Operator1 : RelationalOperator  Operator===  OutDataTypeStr=boolean  InputSameDT=off
  Unit Delay : UnitDelay  SampleTime=-1  HasFrameUpgradeWarning=on
  Q : Outport
  wires:
  Data Type Conversion1/1 -> Relational Operator1/1, Relational Operator/2, Unit Delay/1
  Constant/1 -> Relational Operator1/2
  Logical Operator/1 -> Q/1
  Relational Operator1/1 -> Logical Operator/2
  Relational Operator/1 -> Logical Operator/1
  Unit Delay/1 -> Relational Operator/1
  CLK/1 -> Data Type Conversion1/1

== system Kitchen_Lib/Kitchen/100ms/Kitchn/Subsystem1/Subsystem19/KSW_Battery/BatteryVoltageUnder23V/TimePulse1/TimePulseOriginal/RisingEdgeDetection1 ==
  CLK : Inport
  Constant : Constant  Value=boolean(1)  OutDataTypeStr=boolean
  Data Type Conversion1 : DataTypeConversion  OutDataTypeStr=boolean  SaturateOnIntegerOverflow=off  RndMeth=Floor
  Logical Operator : Logic  AllPortsSameDT=off  OutDataTypeStr=boolean
  Relational Operator : RelationalOperator  Operator=~=  OutDataTypeStr=boolean  InputSameDT=off
  Relational Operator1 : RelationalOperator  Operator===  OutDataTypeStr=boolean  InputSameDT=off
  Unit Delay : UnitDelay  SampleTime=-1  HasFrameUpgradeWarning=on
  Q : Outport
  wires:
  Data Type Conversion1/1 -> Relational Operator1/1, Relational Operator/2, Unit Delay/1
  Constant/1 -> Relational Operator1/2
  Logical Operator/1 -> Q/1
  Relational Operator1/1 -> Logical Operator/2
  Relational Operator/1 -> Logical Operator/1
  Unit Delay/1 -> Relational Operator/1
  CLK/1 -> Data Type Conversion1/1

== system Kitchen_Lib/Kitchen/100ms/Kitchn/Subsystem1/Subsystem19/KSW_Battery/BatteryVoltageUnder23V/TimePulse1/TimePulseOriginal/SR ==
  S : Inport
  R : Inport  Port=2
  Constant1 : Constant  Value=boolean(1)  OutDataTypeStr=boolean
  Constant3 : Constant  Value=boolean(0)  OutDataTypeStr=boolean
  Data Type Conversion1 : DataTypeConversion  OutDataTypeStr=boolean  SaturateOnIntegerOverflow=off  RndMeth=Floor
  Data Type Conversion2 : DataTypeConversion  OutDataTypeStr=boolean  SaturateOnIntegerOverflow=off  RndMeth=Floor
  Multiport Switch : MultiPortSwitch  DataPortOrder=Zero-based contiguous  Inputs=2  zeroidx=on  SaturateOnIntegerOverflow=off  InputSameDT=off
  Multiport Switch1 : MultiPortSwitch  DataPortOrder=Zero-based contiguous  Inputs=2  zeroidx=on  SaturateOnIntegerOverflow=off  InputSameDT=off
  Unit Delay : UnitDelay  SampleTime=-1  HasFrameUpgradeWarning=on
  Q : Outport
  wires:
  Data Type Conversion2/1 -> Multiport Switch/1
  Data Type Conversion1/1 -> Multiport Switch1/1
  Constant3/1 -> Multiport Switch1/3
  Multiport Switch/1 -> Unit Delay/1, Q/1
  Unit Delay/1 -> Multiport Switch1/2
  R/1 -> Data Type Conversion1/1
  Multiport Switch1/1 -> Multiport Switch/2
  Constant1/1 -> Multiport Switch/3
  S/1 -> Data Type Conversion2/1

== system Kitchen_Lib/Kitchen/100ms/Kitchn/Subsystem1/Subsystem19/KSW_Battery/BatteryVoltageUnder23V/TimePulse1/TimePulseOriginal/TimerCountingUpOriginal ==
  TimerEnable : Inport
  TimerReset : Inport  Port=2
  TimerThreshold : Inport  Port=3
  CycleTime : Inport  Port=4
  Data Type Conversion2 : DataTypeConversion  OutDataTypeStr=boolean  SaturateOnIntegerOverflow=off  RndMeth=Floor
  Data Type Conversion4 : DataTypeConversion  OutDataTypeStr=uint32  SaturateOnIntegerOverflow=off  RndMeth=Floor
  Data Type Conversion5 : DataTypeConversion  OutDataTypeStr=uint32  SaturateOnIntegerOverflow=off  RndMeth=Floor
  Data Type Conversion6 : DataTypeConversion  OutDataTypeStr=uint32  SaturateOnIntegerOverflow=off  RndMeth=Floor
  Data Type Conversion7 : DataTypeConversion  OutDataTypeStr=boolean  SaturateOnIntegerOverflow=off  RndMeth=Floor
  Delay : Delay  DelayLength=1  InitialCondition=0  ExternalReset=Rising
      settings: InputPortMap=u0,r5
  Delay1 : Delay  DelayLength=1  InitialCondition=0
  Logical Operator1 : Logic  Operator=NOT  AllPortsSameDT=off  OutDataTypeStr=boolean
  Logical Operator2 : Logic  AllPortsSameDT=off  OutDataTypeStr=boolean
  Logical Operator3 : Logic  Operator=OR  AllPortsSameDT=off  OutDataTypeStr=boolean
  Multiport Switch : MultiPortSwitch  DataPortOrder=Zero-based contiguous  Inputs=2  zeroidx=on  SaturateOnIntegerOverflow=off  InputSameDT=off
  Multiport Switch1 : MultiPortSwitch  DataPortOrder=Zero-based contiguous  Inputs=2  zeroidx=on  SaturateOnIntegerOverflow=off  InputSameDT=off
  Multiport Switch2 : MultiPortSwitch  DataPortOrder=Zero-based contiguous  Inputs=2  zeroidx=on  SaturateOnIntegerOverflow=off  InputSameDT=off
  Relational Operator : RelationalOperator  OutDataTypeStr=boolean  InputSameDT=off
  Relational Operator1 : RelationalOperator  Operator===  OutDataTypeStr=boolean  InputSameDT=off
  RisingEdgeDetection : Subsystem  AncestorBlock=MAN_Library/RisingEdgeDetection
  StartValue_ms1 : Constant  Value=uint32(4294967295)  OutDataTypeStr=uint32
  StartValue_ms2 : Constant  Value=uint32(4294967295)  OutDataTypeStr=uint32
  StartValue_ms3 : Constant  Value=uint32(0)  OutDataTypeStr=uint32
  StartValue_ms5 : Constant  Value=uint32(4294967295)  OutDataTypeStr=uint32
  Sum : Sum
  U32_Saturation : Subsystem  AncestorBlock=MAN_Library/U32_Saturation
  TimerFlag : Outport
  TimerCurrentValue : Outport  Port=2
  wires:
  CycleTime/1 -> Data Type Conversion4/1
  Data Type Conversion2/1 -> Logical Operator3/1
  RisingEdgeDetection/1(Q) -> Logical Operator3/2
  TimerReset/1 -> Data Type Conversion2/1
  TimerEnable/1 -> Data Type Conversion7/1
  Data Type Conversion6/1 -> Relational Operator/2
  Data Type Conversion4/1 -> Sum/2
  StartValue_ms3/1 -> U32_Saturation/3(LowerLimit), Multiport Switch/3
  Multiport Switch2/1 -> U32_Saturation/2(IN)
  Sum/1 -> Multiport Switch2/2
  StartValue_ms2/1 -> Multiport Switch2/3
  Relational Operator1/1 -> Multiport Switch2/1
  Delay/1 -> Multiport Switch1/2, Relational Operator1/1, Sum/1
  StartValue_ms5/1 -> Relational Operator1/2
  Logical Operator3/1 -> Multiport Switch/1, [ResetTimer_BOOL]
  StartValue_ms1/1 -> U32_Saturation/1(UpperLimit)
  Delay1/1 -> Logical Operator1/1
  U32_Saturation/1(OUT) -> Multiport Switch1/3
  Logical Operator1/1 -> Logical Operator2/2
  Logical Operator2/1 -> Multiport Switch1/1
  Data Type Conversion5/1 -> TimerCurrentValue/1, Delay/1, Relational Operator/1
  Data Type Conversion7/1 -> Logical Operator2/1, RisingEdgeDetection/1(CLK)
  Multiport Switch/1 -> Data Type Conversion5/1
  Relational Operator/1 -> TimerFlag/1, Delay1/1
  Multiport Switch1/1 -> Multiport Switch/2
  TimerThreshold/1 -> Data Type Conversion6/1
  [ResetTimer_BOOL] -> Delay/2

== system Kitchen_Lib/Kitchen/100ms/Kitchn/Subsystem1/Subsystem19/KSW_Battery/BatteryVoltageUnder23V/TurnOffDelay/TurnOffDelayOriginal/FallingEdgeDetection ==
  CLK : Inport
  Constant : Constant  Value=boolean(0)  OutDataTypeStr=boolean
  Data Type Conversion1 : DataTypeConversion  OutDataTypeStr=boolean  SaturateOnIntegerOverflow=off  RndMeth=Floor
  Logical Operator1 : Logic  AllPortsSameDT=off  OutDataTypeStr=boolean
  Relational Operator2 : RelationalOperator  Operator=~=  OutDataTypeStr=boolean  InputSameDT=off
  Relational Operator3 : RelationalOperator  Operator===  OutDataTypeStr=boolean  InputSameDT=off
  Unit Delay1 : UnitDelay  SampleTime=-1  HasFrameUpgradeWarning=on
  Q : Outport
  wires:
  Data Type Conversion1/1 -> Unit Delay1/1, Relational Operator2/2, Relational Operator3/1
  Constant/1 -> Relational Operator3/2
  CLK/1 -> Data Type Conversion1/1
  Logical Operator1/1 -> Q/1
  Relational Operator3/1 -> Logical Operator1/2
  Relational Operator2/1 -> Logical Operator1/1
  Unit Delay1/1 -> Relational Operator2/1

== system Kitchen_Lib/Kitchen/100ms/Kitchn/Subsystem1/Subsystem19/KSW_Battery/BatteryVoltageUnder23V/TurnOffDelay/TurnOffDelayOriginal/TimePulseOriginal ==
  TimePulseEnable : Inport
  TimePulseDuration : Inport  Port=2
  CycleTime : Inport  Port=3
  Data Type Conversion1 : DataTypeConversion  OutDataTypeStr=uint32  SaturateOnIntegerOverflow=off  RndMeth=Floor
  Data Type Conversion2 : DataTypeConversion  OutDataTypeStr=boolean  SaturateOnIntegerOverflow=off  RndMeth=Floor
  Delay1 : Delay  DelayLength=1  InitialCondition=0  ExternalReset=Rising
      settings: InputPortMap=u0,r5
  Logical Operator1 : Logic  Operator=NOT  AllPortsSameDT=off  OutDataTypeStr=boolean
  Logical Operator2 : Logic  AllPortsSameDT=off  OutDataTypeStr=boolean
  RisingEdgeDetection : Subsystem  AncestorBlock=MAN_Library/RisingEdgeDetection
  RisingEdgeDetection1 : Subsystem  AncestorBlock=MAN_Library/RisingEdgeDetection
  SR : Subsystem  AncestorBlock=MAN_Library/SR
  TimerCountingUpOriginal : Subsystem  AncestorBlock=MAN_Library/BasicLibrary/TimerCountingUpOriginal
  TimePulseFlag : Outport
  TimePulseExpiredTime : Outport  Port=2
  wires:
  CycleTime/1 -> TimerCountingUpOriginal/4(CycleTime)
  Delay1/1 -> SR/2(R)
  [TimePulseReset] -> TimerCountingUpOriginal/2(TimerReset)
  [TimePulseReset] -> Delay1/2
  RisingEdgeDetection/1(Q) -> SR/1(S), [TimePulseReset]
  Data Type Conversion1/1 -> TimerCountingUpOriginal/3(TimerThreshold)
  Data Type Conversion2/1 -> RisingEdgeDetection/1(CLK)
  Logical Operator1/1 -> Logical Operator2/2
  Logical Operator2/1 -> TimePulseFlag/1
  RisingEdgeDetection1/1(Q) -> Delay1/1
  TimerCountingUpOriginal/1(TimerFlag) -> RisingEdgeDetection1/1(CLK), Logical Operator1/1
  SR/1(Q) -> Logical Operator2/1, TimerCountingUpOriginal/1(TimerEnable)
  TimePulseEnable/1 -> Data Type Conversion2/1
  TimePulseDuration/1 -> Data Type Conversion1/1
  TimerCountingUpOriginal/2(TimerCurrentValue) -> TimePulseExpiredTime/1

== system Kitchen_Lib/Kitchen/100ms/Kitchn/Subsystem1/Subsystem19/KitchenEnable/KitchenOffAutomaticIgnitionOff/TurnOnDelay/TurnOnDelayOriginal/RisingEdgeDetection ==
  CLK : Inport
  Constant : Constant  Value=boolean(1)  OutDataTypeStr=boolean
  Data Type Conversion1 : DataTypeConversion  OutDataTypeStr=boolean  SaturateOnIntegerOverflow=off  RndMeth=Floor
  Logical Operator : Logic  AllPortsSameDT=off  OutDataTypeStr=boolean
  Relational Operator : RelationalOperator  Operator=~=  OutDataTypeStr=boolean  InputSameDT=off
  Relational Operator1 : RelationalOperator  Operator===  OutDataTypeStr=boolean  InputSameDT=off
  Unit Delay : UnitDelay  SampleTime=-1  HasFrameUpgradeWarning=on
  Q : Outport
  wires:
  Data Type Conversion1/1 -> Relational Operator1/1, Relational Operator/2, Unit Delay/1
  Constant/1 -> Relational Operator1/2
  Logical Operator/1 -> Q/1
  Relational Operator1/1 -> Logical Operator/2
  Relational Operator/1 -> Logical Operator/1
  Unit Delay/1 -> Relational Operator/1
  CLK/1 -> Data Type Conversion1/1

== system Kitchen_Lib/Kitchen/100ms/Kitchn/Subsystem1/Subsystem19/KitchenEnable/KitchenOffAutomaticIgnitionOff/TurnOnDelay/TurnOnDelayOriginal/TimePulseOriginal ==
  TimePulseEnable : Inport
  TimePulseDuration : Inport  Port=2
  CycleTime : Inport  Port=3
  Data Type Conversion1 : DataTypeConversion  OutDataTypeStr=uint32  SaturateOnIntegerOverflow=off  RndMeth=Floor
  Data Type Conversion2 : DataTypeConversion  OutDataTypeStr=boolean  SaturateOnIntegerOverflow=off  RndMeth=Floor
  Delay1 : Delay  DelayLength=1  InitialCondition=0  ExternalReset=Rising
      settings: InputPortMap=u0,r5
  Logical Operator1 : Logic  Operator=NOT  AllPortsSameDT=off  OutDataTypeStr=boolean
  Logical Operator2 : Logic  AllPortsSameDT=off  OutDataTypeStr=boolean
  RisingEdgeDetection : Subsystem  AncestorBlock=MAN_Library/RisingEdgeDetection
  RisingEdgeDetection1 : Subsystem  AncestorBlock=MAN_Library/RisingEdgeDetection
  SR : Subsystem  AncestorBlock=MAN_Library/SR
  TimerCountingUpOriginal : Subsystem  AncestorBlock=MAN_Library/BasicLibrary/TimerCountingUpOriginal
  TimePulseFlag : Outport
  TimePulseExpiredTime : Outport  Port=2
  wires:
  CycleTime/1 -> TimerCountingUpOriginal/4(CycleTime)
  Delay1/1 -> SR/2(R)
  [TimePulseReset] -> TimerCountingUpOriginal/2(TimerReset)
  [TimePulseReset] -> Delay1/2
  RisingEdgeDetection/1(Q) -> SR/1(S), [TimePulseReset]
  Data Type Conversion1/1 -> TimerCountingUpOriginal/3(TimerThreshold)
  Data Type Conversion2/1 -> RisingEdgeDetection/1(CLK)
  Logical Operator1/1 -> Logical Operator2/2
  Logical Operator2/1 -> TimePulseFlag/1
  RisingEdgeDetection1/1(Q) -> Delay1/1
  TimerCountingUpOriginal/1(TimerFlag) -> RisingEdgeDetection1/1(CLK), Logical Operator1/1
  SR/1(Q) -> Logical Operator2/1, TimerCountingUpOriginal/1(TimerEnable)
  TimePulseEnable/1 -> Data Type Conversion2/1
  TimePulseDuration/1 -> Data Type Conversion1/1
  TimerCountingUpOriginal/2(TimerCurrentValue) -> TimePulseExpiredTime/1

== system Kitchen_Lib/Kitchen/100ms/Kitchn/Subsystem1/Subsystem19/KitchenEnable/Subsystem/TurnOnDelay/TurnOnDelayOriginal/RisingEdgeDetection ==
  CLK : Inport
  Constant : Constant  Value=boolean(1)  OutDataTypeStr=boolean
  Data Type Conversion1 : DataTypeConversion  OutDataTypeStr=boolean  SaturateOnIntegerOverflow=off  RndMeth=Floor
  Logical Operator : Logic  AllPortsSameDT=off  OutDataTypeStr=boolean
  Relational Operator : RelationalOperator  Operator=~=  OutDataTypeStr=boolean  InputSameDT=off
  Relational Operator1 : RelationalOperator  Operator===  OutDataTypeStr=boolean  InputSameDT=off
  Unit Delay : UnitDelay  SampleTime=-1  HasFrameUpgradeWarning=on
  Q : Outport
  wires:
  Data Type Conversion1/1 -> Relational Operator1/1, Relational Operator/2, Unit Delay/1
  Constant/1 -> Relational Operator1/2
  Logical Operator/1 -> Q/1
  Relational Operator1/1 -> Logical Operator/2
  Relational Operator/1 -> Logical Operator/1
  Unit Delay/1 -> Relational Operator/1
  CLK/1 -> Data Type Conversion1/1
